simulink model "Linear_Model_Check_mks_4Nov"  (R2022b)
settings: Solver=VariableStepAuto  StartTime=0.0  StopTime=10000  FixedStep=0.5  RelTol=1e-6
settings Model: Creator=Mitarbeiter  LastModifiedBy=Mitarbeiter

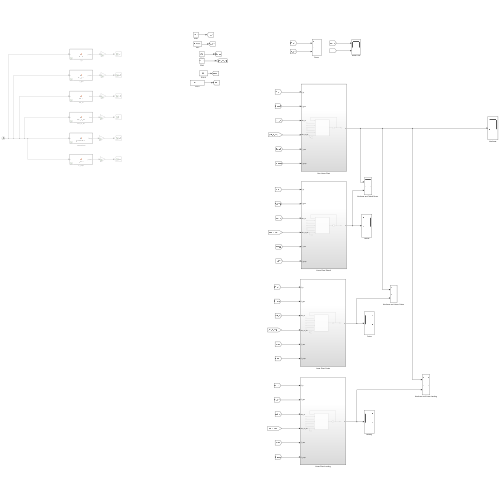
[thumbnail: Simulink's stored preview of the top-level diagram]
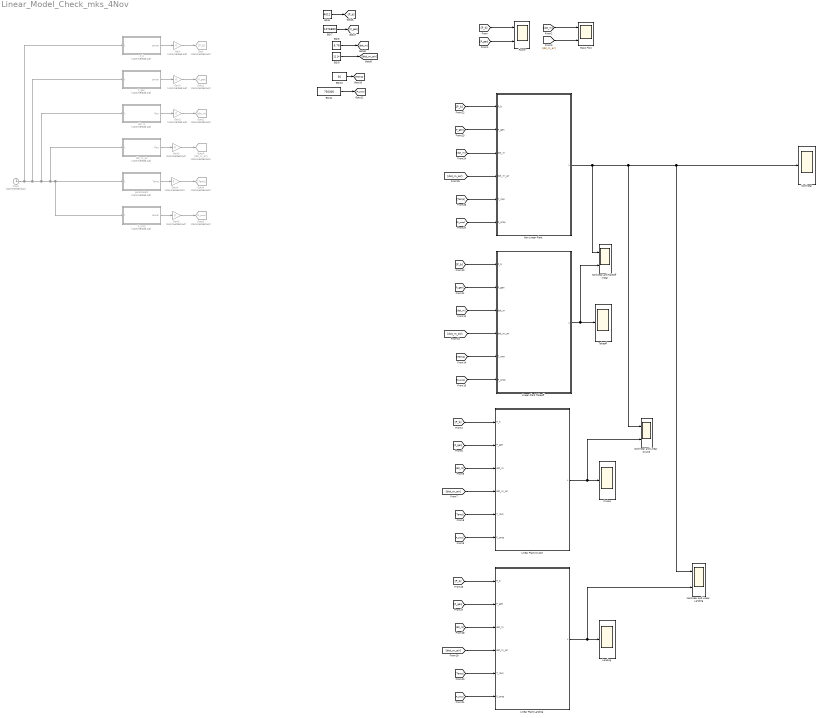
== system Linear_Model_Check_mks_4Nov ==
  Clock : Clock  Commented=on
  Cruise : Scope
  EQI10 : Constant  Value=30
  EQI11 : Constant  Value=750000
  EQI6 : Constant  Value=4012  SampleTime=-1
  EQI7 : Constant  Value=1076880
  EQI8 : Constant  Value=6.76
  EQI9 : Constant  Value=12.14
  Gain{,1..5} (6 alike) : Gain  Commented=on  Gain=0
  Goto : Goto  Commented=on  GotoTag=P_b
  Goto1 : Goto  Commented=on  GotoTag=P_gen
  Goto2 : Goto  Commented=on  GotoTag=dot_m
  Goto3 : Goto  Commented=on  GotoTag=dot_m_air
  Goto4 : Goto  Commented=on  GotoTag=Temp
  Goto5 : Goto  Commented=on  GotoTag=P_prop
  Landing : Scope
  Linear Plant Cruise : Subsystem
  Linear Plant Landing : Subsystem
  Linear Plant Takeoff : Subsystem
  Mass Flow : Scope  NumInputPorts=2
  Non Linear Plant : Subsystem
  Nonlinear : Scope
  Nonlinear and Linear Cruise : Scope  NumInputPorts=2
  Nonlinear and Linear Landing : Scope  NumInputPorts=2
  "Nonlinear and Takeoff linear " : Scope  NumInputPorts=2
  P_b : MATLAB Function  Commented=on  TreatAsAtomicUnit=on
  P_gen : MATLAB Function  Commented=on  TreatAsAtomicUnit=on
  P_prop : MATLAB Function  Commented=on  TreatAsAtomicUnit=on
  Power : Scope  NumInputPorts=2
  Takeoff : Scope
  dot_m : MATLAB Function  Commented=on  TreatAsAtomicUnit=on
  dot_m_air : MATLAB Function  Commented=on  TreatAsAtomicUnit=on
  parameters : MATLAB Function  Commented=on  TreatAsAtomicUnit=on
  wires:
  [P_b] -> Power/1
  [P_gen] -> Power/2
  [dot_m] -> Mass Flow/1
  [dot_m_air] -> Mass Flow/2
  EQI6/1 -> [P_b]
  EQI7/1 -> [P_gen]
  EQI8/1 -> [dot_m]
  EQI9/1 -> [dot_m_air]
  EQI10/1 -> [Temp]
  EQI11/1 -> [P_prop]
  [Temp] -> Linear Plant Takeoff/5(T_ram)
  [P_prop] -> Linear Plant Takeoff/6(P_prop)
  [dot_m_air] -> Linear Plant Takeoff/4(dot_m_air)
  [P_gen] -> Linear Plant Takeoff/2(P_gen)
  [P_b] -> Linear Plant Takeoff/1(P_b)
  Linear Plant Takeoff/1(x) -> Takeoff/1, "Nonlinear and Takeoff linear "/2
  [dot_m] -> Linear Plant Takeoff/3(dot_m)
  [P_b] -> Linear Plant Cruise/1(P_b)
  [dot_m] -> Linear Plant Cruise/3(dot_m)
  Linear Plant Cruise/1(x) -> Nonlinear and Linear Cruise/2, Cruise/1
  [Temp] -> Linear Plant Cruise/5(T_ram)
  [P_prop] -> Linear Plant Cruise/6(P_prop)
  [dot_m_air] -> Linear Plant Cruise/4(dot_m_air)
  [P_gen] -> Linear Plant Cruise/2(P_gen)
  [P_gen] -> Linear Plant Landing/2(P_gen)
  [dot_m_air] -> Linear Plant Landing/4(dot_m_air)
  [P_b] -> Linear Plant Landing/1(P_b)
  [P_prop] -> Linear Plant Landing/6(P_prop)
  [dot_m] -> Linear Plant Landing/3(dot_m)
  Linear Plant Landing/1(x) -> Nonlinear and Linear Landing/2, Landing/1
  [Temp] -> Linear Plant Landing/5(T_ram)
  Gain5/1 -> Goto5/1
  P_b/1(power) -> Gain/1
  Gain2/1 -> Goto2/1
  Gain/1 -> Goto/1
  Gain1/1 -> Goto1/1
  P_gen/1(power) -> Gain1/1
  Gain3/1 -> Goto3/1
  P_prop/1(power) -> Gain5/1
  parameters/1(Temp) -> Gain4/1
  Clock/1 -> P_b/1(t), P_gen/1(t), dot_m/1(t), dot_m_air/1(t), parameters/1(t), P_prop/1(t)
  Gain4/1 -> Goto4/1
  dot_m/1(flow) -> Gain2/1
  dot_m_air/1(flow) -> Gain3/1
  [P_b] -> Non Linear Plant/1(P_b)
  [dot_m] -> Non Linear Plant/3(dot_m)
  Non Linear Plant/1(x) -> Nonlinear and Linear Cruise/1, Nonlinear and Linear Landing/1, Nonlinear/1, "Nonlinear and Takeoff linear "/1
  [Temp] -> Non Linear Plant/5(T_ram)
  [P_prop] -> Non Linear Plant/6(P_prop)
  [dot_m_air] -> Non Linear Plant/4(dot_m_air)
  [P_gen] -> Non Linear Plant/2(P_gen)

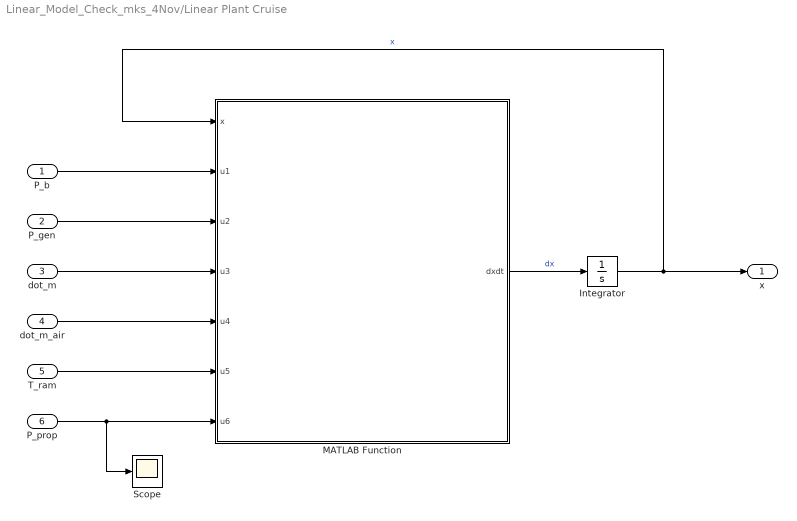
== system Linear_Model_Check_mks_4Nov/Linear Plant Cruise ==
  P_b : Inport
  P_gen : Inport  Port=2
  dot_m : Inport  Port=3
  dot_m_air : Inport  Port=4
  T_ram : Inport  Port=5
  P_prop : Inport  Port=6
  Integrator : Integrator  InitialCondition=[52814776030872794621339/2111078349043945281000; 104094200346052350023/4282106184673317000; 0.95; 7429519190417529794477/301582621291992183000; 14970426814841764289/611729454953331000; 62413813461003262061339/2111078349043945281000; 115709353125739950023/4282106184673317000; 1317031521595249/55809639171000; 192210910256741628225757/6125247032447703303000; 18157083865504564289/611729454953331000; 1317031521595249/55809639171000; 29037669531913/1240214203800; 1405698391771/60204573000];
  MATLAB Function : MATLAB Function  TreatAsAtomicUnit=on
  Scope : Scope
  x : Outport
  wires:
  MATLAB Function/1(dxdt) -> Integrator/1  "dx"
  Integrator/1 -> x/1, MATLAB Function/1(x)  "x"
  P_prop/1 -> Scope/1, MATLAB Function/7(u6)
  P_b/1 -> MATLAB Function/2(u1)
  P_gen/1 -> MATLAB Function/3(u2)
  dot_m/1 -> MATLAB Function/4(u3)
  dot_m_air/1 -> MATLAB Function/5(u4)
  T_ram/1 -> MATLAB Function/6(u5)

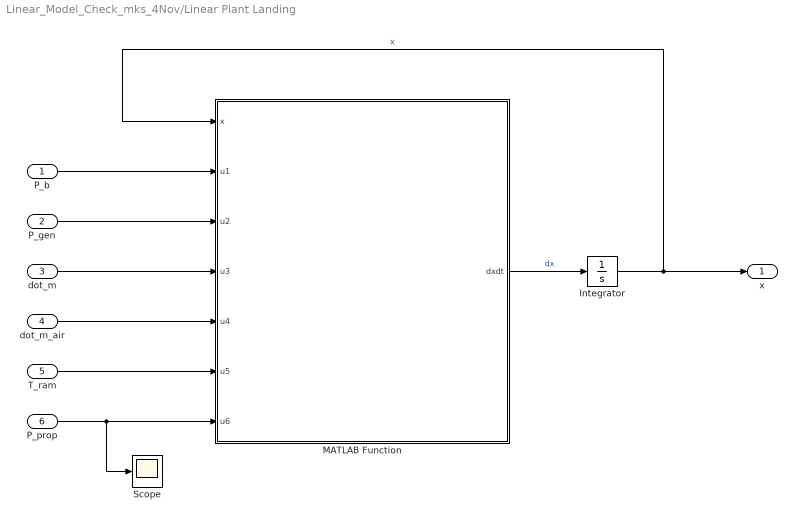
== system Linear_Model_Check_mks_4Nov/Linear Plant Landing ==
  P_b : Inport
  P_gen : Inport  Port=2
  dot_m : Inport  Port=3
  dot_m_air : Inport  Port=4
  T_ram : Inport  Port=5
  P_prop : Inport  Port=6
  Integrator : Integrator  InitialCondition=[93988057444394599308387229/4422589792359066198000000; 14175896344014406900981/690059259222822000000; 0.95; 642296550198010131218710603/30958128546513463386000000; 99794188918686328306867/4830414814559754000000; 748871653711516104483208603/30958128546513463386000000; 109523475430206270118867/4830414814559754000000; 114489338227757388521/5840888530302000000; 1232797079008717771442215271/48366943538186816802000000; 118698981952749594118867/4830414814559754000000; 114489338227757388521/5840888530302000000; 1053909433374709813/54082301206500000; 8752431102689/450060759000]
  MATLAB Function : MATLAB Function  TreatAsAtomicUnit=on
  Scope : Scope
  x : Outport
  wires:
  MATLAB Function/1(dxdt) -> Integrator/1  "dx"
  Integrator/1 -> x/1, MATLAB Function/1(x)  "x"
  P_prop/1 -> Scope/1, MATLAB Function/7(u6)
  P_b/1 -> MATLAB Function/2(u1)
  P_gen/1 -> MATLAB Function/3(u2)
  dot_m/1 -> MATLAB Function/4(u3)
  dot_m_air/1 -> MATLAB Function/5(u4)
  T_ram/1 -> MATLAB Function/6(u5)

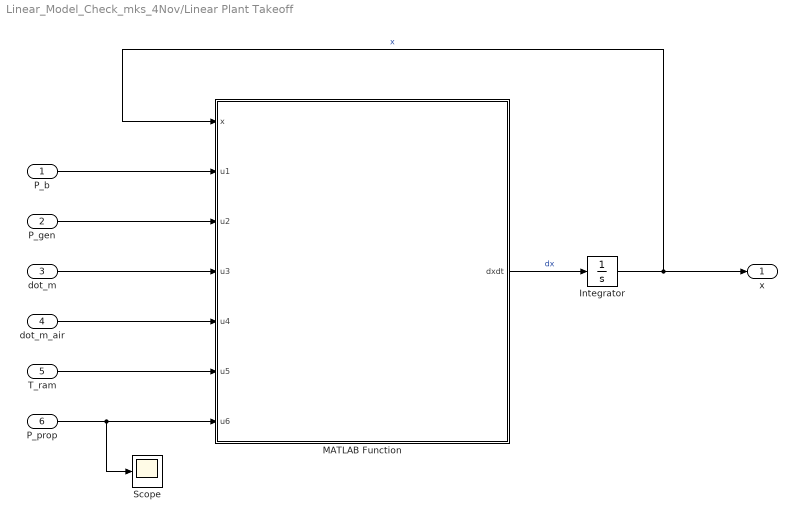
== system Linear_Model_Check_mks_4Nov/Linear Plant Takeoff ==
  P_b : Inport
  P_gen : Inport  Port=2
  dot_m : Inport  Port=3
  dot_m_air : Inport  Port=4
  T_ram : Inport  Port=5
  P_prop : Inport  Port=6
  Integrator : Integrator  InitialCondition=[20275100030210626643675627/393605954186145082200000; 2979945209973437579603/61414566107995800000; 0.95; 19353199461943751447675627/393605954186145082200000; 3002556108225437579603/61414566107995800000; 21715964372172979203125627/393605954186145082200000; 3222032306869374239603/61414566107995800000; 657622429946024881/14752478046600000; 37742600191627471661144839/614944050439361945400000; 3590589948376974239603/61414566107995800000; 657622429946024881/14752478046600000; 81610506679008893/1844059755825000; 9032287404091/204611346000]
  MATLAB Function : MATLAB Function  TreatAsAtomicUnit=on
  Scope : Scope
  x : Outport
  wires:
  MATLAB Function/1(dxdt) -> Integrator/1  "dx"
  Integrator/1 -> x/1, MATLAB Function/1(x)  "x"
  P_prop/1 -> Scope/1, MATLAB Function/7(u6)
  P_b/1 -> MATLAB Function/2(u1)
  P_gen/1 -> MATLAB Function/3(u2)
  dot_m/1 -> MATLAB Function/4(u3)
  dot_m_air/1 -> MATLAB Function/5(u4)
  T_ram/1 -> MATLAB Function/6(u5)

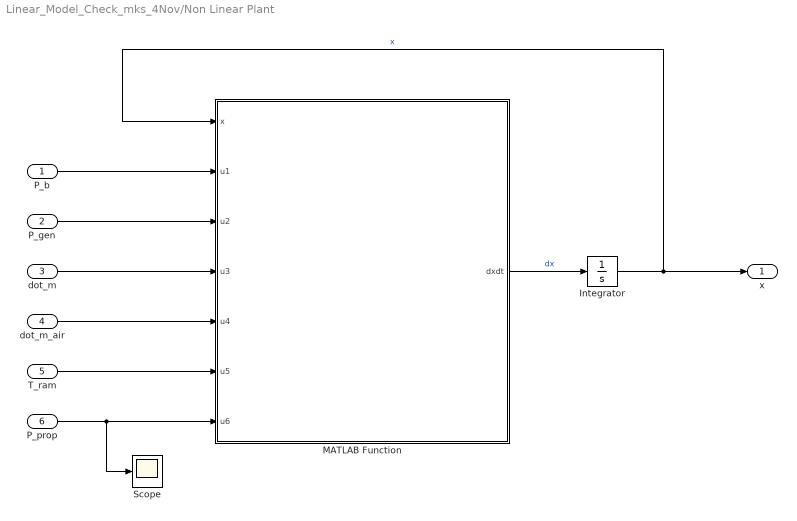
== system Linear_Model_Check_mks_4Nov/Non Linear Plant ==
  P_b : Inport
  P_gen : Inport  Port=2
  dot_m : Inport  Port=3
  dot_m_air : Inport  Port=4
  T_ram : Inport  Port=5
  P_prop : Inport  Port=6
  Integrator : Integrator  InitialCondition=[93988057444394599308387229/4422589792359066198000000; 14175896344014406900981/690059259222822000000; 0.95; 642296550198010131218710603/30958128546513463386000000; 99794188918686328306867/4830414814559754000000; 20; 748871653711516104483208603/30958128546513463386000000; 109523475430206270118867/4830414814559754000000; 20; 114489338227757388521/5840888530302000000; 20; 1232797079008717771442215271/48366943538186816802000000; 118698981952749594118867/4830414814559754000000; 114489338227757388521/5840888530302000000; 1053909433374709813/54082301206500000; 8752431102689/450060759000]
  MATLAB Function : MATLAB Function  TreatAsAtomicUnit=on
  Scope : Scope
  x : Outport
  wires:
  MATLAB Function/1(dxdt) -> Integrator/1  "dx"
  Integrator/1 -> x/1, MATLAB Function/1(x)  "x"
  P_prop/1 -> Scope/1, MATLAB Function/7(u6)
  P_b/1 -> MATLAB Function/2(u1)
  P_gen/1 -> MATLAB Function/3(u2)
  dot_m/1 -> MATLAB Function/4(u3)
  dot_m_air/1 -> MATLAB Function/5(u4)
  T_ram/1 -> MATLAB Function/6(u5)

== matlab function Linear_Model_Check_mks_4Nov/parameters ==
  data: t input; Temp output
function Temp  = parameters(t)
    %% Calculates aircraft altitude in ft and m

    T_off = 60;
    cruise_t = 1380;
    landing_t = 3240;
    final_t = 4500;

    slope1 = 0.25/T_off; % 0.25 / 1
    slope2 = (0.4 - 0.25) / (cruise_t - T_off);
    slope3 = (0.25 - 0.4) / (final_t - landing_t);

    ramp = zeros(size(t));
    ramp(t <= T_off) = slope1 * t(t <= T_off);
    
    ramp1 = zeros(size(t));
    ramp1(t > T_off & t < cruise_t) = slope2 * (t(t > T_off & t < cruise_t) - T_off) + 0.25;
    
    ramp2 = zeros(size(t));
    ramp2(t >= cruise_t & t <= landing_t) = 0.4;
    
    ramp3 = zeros(size(t));
    ramp3(t > landing_t & t <= 4500) = slope3 * (t(t > landing_t & t <= 4500) - landing_t) + 0.4;
    
    ramp4 = zeros(size(t));
    ramp4(t > 4500) = slope3 * (t(t > 4500) - 4500) + 0.25;
    
    Speed = ramp + ramp1 + ramp2 + ramp3 + ramp4;

    %% T_ram calculations
    r_slope1 = 0;
    r_slope2 = (-35 - 30) / (1380 - 60);
    r_slope3 = 0;
    
    r_slope5 = (30 - (-35)) / (4500 - 3240);
    
    Gamma = 1.4;
    
    ramp = zeros(size(t));
    ramp(t <= T_off) = r_slope1 * t(t <= T_off) + 30;
    
    ramp1 = zeros(size(t));
    ramp1(t > T_off & t < cruise_t) = r_slope2 * (t(t > T_off & t < cruise_t) - T_off) + 30;
    
    ramp2 = zeros(size(t));
    ramp2(t >= cruise_t & t <= landing_t) = -35;
    
    ramp3 = zeros(size(t));
    ramp3(t > landing_t & t <= 4500) = r_slope5 * (t(t > landing_t & t <= 4500) - landing_t) - 35;
    
    ramp4 = zeros(size(t));
    ramp4(t > 4500) = r_slope3 * (t(t > 4500) - 4500) + 30;
    
    T_amp = ramp + ramp1 + ramp2 + ramp3 + ramp4;

     Temp = T_amp.*(1+Speed.^2 * ((Gamma-1)/2));
%     Temp = 30 * ones(size(t));

end

== matlab function Linear_Model_Check_mks_4Nov/Linear Plant Cruise/MATLAB Function ==
  data: x input; dxdt output; u1 input; u2 input; u3 input; u4 input; u5 input; u6 input
function dxdt = fcn(x,u1,u2,u3,u4,u5,u6)

u = [u1;u2;u3;u4;u5;u6];
dxdt = aircraft_dynamics_linear_cruise(x,u);

== matlab function Linear_Model_Check_mks_4Nov/Linear Plant Landing/MATLAB Function ==
  data: x input; dxdt output; u1 input; u2 input; u3 input; u4 input; u5 input; u6 input
function dxdt = fcn(x,u1,u2,u3,u4,u5,u6)

u = [u1;u2;u3;u4;u5;u6];
dxdt = aircraft_dynamics_linear_landing(x,u);

== matlab function Linear_Model_Check_mks_4Nov/P_b ==
  data: t input; power output
function power = P_b(t)
    % Define the power values vector
    power_values = [541728.972461324, 525434.547259656, 484698.484257782, ...
                    443962.421182278, 403226.358083855, 362490.295190934, ...
                    321754.232292711, 281018.169380235, 240282.106417171, ...
                    199546.043463649, 158809.980492022, 118073.917524794, ...
                    77337.8545513178, 36601.7915815174, 4012.94120061964, ...
                    4012.94120060897, 4012.94120058611, 4012.94120055903, ...
                    4012.94120053569, 4012.94120052215, 4012.94120051169, ...
                    4012.94120050506, 4012.94120050103, 4012.94120049878, ...
                    4012.94120049977, 4012.94120050145, 4012.94120050538, ...
                    4012.94120051198, 4012.94120052045, 4012.94120053546, ...
                    4012.94120055757, 4012.94120058035, 4012.94120057094, ...
                    9.73312208790910e-10, -3.25790856001986e-10, ...
                    -7.33764827360896e-10, -3.22870604452897e-11, ...
                    -2.89901400312855e-11, -6.19593223381754e-11, ...
                    -4.77143652162351e-10, 3.07295526727322e-10, ...
                    -5.97594860992170e-10, 7.70455739254353e-10, ...
                    -4.62243586863996e-11, 65143.2880368747];

    % Define the corresponding time vector (every 10 seconds from 0 to 4500)
    time_vector = 1:100:4500;

    % Check if input t is within the range of 0 to 4500
    if t < 0 || t > 4500
        error('Input time t must be within the range 0 to 4500 seconds.');
    end

    % Create the spline interpolation function
    spline_fit = spline(time_vector, power_values);

    % Evaluate the spline at the desired continuous time t
    power = ppval(spline_fit, t);

%     power = 4012* ones(size(t));
end

== matlab function Linear_Model_Check_mks_4Nov/P_gen ==
  data: t input; power output
function power = P_gen(t)
  
    power_values = [1560823.08194895	1546158.09929008	1509495.64264034	1472833.18607241	1436170.72952995	1399508.27275915	1362845.81599425	1326183.35924518	1289520.90255232	1252858.44584885	1216195.98916551	1179533.53247727	1142871.07579598	1106208.61911061	1076878.65376792	1076878.65376794	1076878.65376796	1076878.65376799	1076878.65376802	1076878.65376803	1076878.65376804	1076878.65376805	1076878.65376806	1076878.65376806	1076878.65376806	1076878.65376806	1076878.65376805	1076878.65376804	1076878.65376803	1076878.65376802	1076878.65376799	1076878.65376797	1076878.65376798	1032182.62799974	950257.879125699	868333.130251657	786408.381377613	704483.632503570	622558.883629528	540634.134755485	458709.385881442	376784.637007400	294859.888133355	212935.139259313	58628.9592331873];
 % Define the corresponding time vector (every 10 seconds from 0 to 4500)
    time_vector = 1:100:4500;

    % Check if input t is within the range of 0 to 4500
    if t < 0 || t > 4500
        error('Input time t must be within the range 0 to 4500 seconds.');
    end

    % Create the spline interpolation function
    spline_fit = spline(time_vector, power_values);

    % Evaluate the spline at the desired continuous time t
    power = ppval(spline_fit, t);

% power = 1076880* ones(size(t));
end

== matlab function Linear_Model_Check_mks_4Nov/P_prop ==
  data: t input; power output
function power = P_prop(t)
    slope = 568.2;
    T_off = 60;
    cruise_t = 1380; % 23min
    landing_t = 3240; % 54min
    step = 1500e3;
    
    ramp1 = zeros(size(t));
    ramp1(t >= T_off) = -slope * (t(t >= T_off) - T_off);
    
    ramp2 = zeros(size(t));
    ramp2(t >= cruise_t) = slope * (t(t >= cruise_t) - cruise_t);
    
    ramp3 = zeros(size(t));
    ramp3(t >= landing_t) = -slope * (t(t >= landing_t) - landing_t);
    
    power = step + ramp1 + ramp2 + ramp3;
    power(power < 0) = 0;
   % power = 750000* ones(size(t));
end

== matlab function Linear_Model_Check_mks_4Nov/dot_m ==
  data: t input; flow output
function flow = dot_m(t)
    % Define the power values vector
    power_values = [0.904165131160427	1.62335959482857	1.97415345554372	2.87737856692485	3.93386755649844	4.17049006426838	3.96224826445125	3.84633136696794	3.73843209854831	3.62816620139765	3.51470105395037	3.39795514134232	3.27785630468602	3.15345777233773	3.04616198439548	3.03635175832522	2.98312074354866	2.91947217209040	2.86878591164222	2.83212849923799	2.80518126603719	2.78469068203536	2.76888505493890	2.75675815114367	2.74763217287481	2.74096591488524	2.73636304275517	2.73354386559958	2.73235420493226	2.73274273164412	2.73475441155951	2.73847704472223	2.74398498698495	2.64313697414983	2.45549965647436	2.26040185709996	2.23930438794837	1.99924539905101	1.61176185199414	1.31895743051123	1.30916014023536	1.07782805041202	0.848496416787671	0.620762639063214	-5.77778983316171e-34];

    % Define the corresponding time vector (every 10 seconds from 0 to 4500)
    time_vector = 1:100:4500;

    % Check if input t is within the range of 0 to 4500
    if t < 0 || t > 4500
        error('Input time t must be within the range 0 to 4500 seconds.');
    end

    % Create the spline interpolation function
    spline_fit = spline(time_vector, power_values);

    % Evaluate the spline at the desired continuous time t
    flow = ppval(spline_fit, t);

%     flow = 6.76* ones(size(t));
end

== matlab function Linear_Model_Check_mks_4Nov/Linear Plant Takeoff/MATLAB Function ==
  data: x input; dxdt output; u1 input; u2 input; u3 input; u4 input; u5 input; u6 input
function dxdt = fcn(x,u1,u2,u3,u4,u5,u6)

u = [u1;u2;u3;u4;u5;u6];
dxdt = aircraft_dynamics_linear_takeoff(x,u);

== matlab function Linear_Model_Check_mks_4Nov/dot_m_air ==
  data: t input; flow output
function flow = dot_m_air(t)
    % Define the power values vector
    power_values = [0.370775472872228	4.14655917085228	10.2236066715828	15.9335661862365	19.0351731908349	16.9149763039733	13.1623042033400	10.7569435504486	8.94905877526484	7.51589529502896	6.36393337822089	5.39660249912924	4.60743235399543	4.39417963045294	4.45647923355531	4.36949731785185	4.31573725145724	4.26746478317914	4.22732179826729	4.19595415374334	4.17143491891122	4.15169555274063	4.13523300363972	4.12099504031059	4.10816091872904	4.09600581489035	4.08381103149970	4.07079463660703	4.05616667450225	4.03954164705557	4.02160559806096	4.00355147248531	3.98237533346872	3.81444977989844	3.58043631849297	3.43750882096772	3.44017594340288	3.48343898919501	3.38952732636595	3.08055145207970	2.48510068273254	1.52973911636135	0.577892294612315	0.0671525631123886	1.01083847375133e-34];

    % Define the corresponding time vector (every 10 seconds from 0 to 4500)
    time_vector = 1:100:4500;

    % Check if input t is within the range of 0 to 4500
    if t < 0 || t > 4500
        error('Input time t must be within the range 0 to 4500 seconds.');
    end

    % Create the spline interpolation function
    spline_fit = spline(time_vector, power_values);

    % Evaluate the spline at the desired continuous time t
    flow = ppval(spline_fit, t);
%     flow = 12.14* ones(size(t));
end

== matlab function Linear_Model_Check_mks_4Nov/Non Linear Plant/MATLAB Function ==
  data: x input; dxdt output; u1 input; u2 input; u3 input; u4 input; u5 input; u6 input
function dxdt = fcn(x,u1,u2,u3,u4,u5,u6)

u = [u1;u2;u3;u4;u5;u6];
dxdt = aircraftDynamicsCT(x,u);
